simulink model "normal_wave_architecture_constant_passive"  (R2021b)
settings: Solver=ode45  StartTime=0.0  StopTime=20  RelTol=1e-5
values from neighbouring files (symbols this model uses):
  b = 2.1    [normal_wave_architecture_constant_parameters.m]    (also in normal_wave_architecture_constant_parameters.m.m = 8.5; normal_wave_architecture_variable_parameters.m = 1; obs_m.m = block.InputPort(3).Data; obs_s.m = block.InputPort(3).Data)
  Be = 5    [normal_wave_architecture_constant_parameters.m]    (also in normal_wave_architecture_constant_parameters.m.m; normal_wave_architecture_variable_parameters.m)
  beta_m = 2*pi*Fc_vel*Ts    (= 0.0628318530718)    [normal_wave_architecture_constant_parameters.m]    (also in normal_wave_architecture_constant_parameters.m.m; normal_wave_architecture_variable_parameters.m)
  beta_s = 2*pi*Fc_vel*Ts    (= 0.0628318530718)    [normal_wave_architecture_constant_parameters.m]    (also in normal_wave_architecture_constant_parameters.m.m; normal_wave_architecture_variable_parameters.m)
  Bh = 0.02    [normal_wave_architecture_constant_parameters.m]    (also in normal_wave_architecture_constant_parameters.m.m; normal_wave_architecture_variable_parameters.m)
  d_m2s = 1    [normal_wave_architecture_constant_parameters.m]    (also in normal_wave_architecture_constant_parameters.m.m = 10; normal_wave_architecture_variable_parameters.m = 0.001)
  d_s2m = 1    [normal_wave_architecture_constant_parameters.m]    (also in normal_wave_architecture_constant_parameters.m.m = 10; normal_wave_architecture_variable_parameters.m = 0.001)
  delta = 1    [normal_wave_architecture_constant_parameters.m]    (also in normal_wave_architecture_constant_parameters.m.m; normal_wave_architecture_variable_parameters.m)
  eQ_m = 2*pi/4096    (= 0.00153398078789)    [normal_wave_architecture_constant_parameters.m]    (also in normal_wave_architecture_constant_parameters.m.m; normal_wave_architecture_variable_parameters.m)
  eQ_s = 2*pi/4096    (= 0.00153398078789)    [normal_wave_architecture_constant_parameters.m]    (also in normal_wave_architecture_constant_parameters.m.m; normal_wave_architecture_variable_parameters.m)
  Fc_h = 5    [normal_wave_architecture_constant_parameters.m]    (also in normal_wave_architecture_constant_parameters.m.m; normal_wave_architecture_variable_parameters.m)
  Filter = 50    [normal_wave_architecture_constant_parameters.m]    (also in normal_wave_architecture_constant_parameters.m.m = 10; normal_wave_architecture_variable_parameters.m = 1)
  Jh = 0.02    [normal_wave_architecture_constant_parameters.m]    (also in normal_wave_architecture_constant_parameters.m.m; normal_wave_architecture_variable_parameters.m)
  k_m = 19.34    [normal_wave_architecture_constant_parameters.m]    (also in normal_wave_architecture_constant_parameters.m.m; normal_wave_architecture_variable_parameters.m)
  k_s = 19.34    [normal_wave_architecture_constant_parameters.m]    (also in normal_wave_architecture_constant_parameters.m.m; normal_wave_architecture_variable_parameters.m)
  Kc2v_m = 4.5    [normal_wave_architecture_constant_parameters.m]    (also in normal_wave_architecture_constant_parameters.m.m; normal_wave_architecture_variable_parameters.m)
  Kc2v_s = 4.5    [normal_wave_architecture_constant_parameters.m]    (also in normal_wave_architecture_constant_parameters.m.m; normal_wave_architecture_variable_parameters.m)
  Kd_h = 0.5    [normal_wave_architecture_constant_parameters.m]    (also in normal_wave_architecture_constant_parameters.m.m; normal_wave_architecture_variable_parameters.m)
  Kd_m = 0.5    [normal_wave_architecture_constant_parameters.m]    (also in normal_wave_architecture_constant_parameters.m.m; normal_wave_architecture_variable_parameters.m)
  Kd_s = 0.5    [normal_wave_architecture_constant_parameters.m]    (also in normal_wave_architecture_constant_parameters.m.m; normal_wave_architecture_variable_parameters.m)
  Ke = 10    [normal_wave_architecture_constant_parameters.m]    (also in normal_wave_architecture_constant_parameters.m.m; normal_wave_architecture_variable_parameters.m)
  Kp_h = 1.2    [normal_wave_architecture_constant_parameters.m]    (also in normal_wave_architecture_constant_parameters.m.m; normal_wave_architecture_variable_parameters.m)
  Kp_m = 1    [normal_wave_architecture_constant_parameters.m]    (also in normal_wave_architecture_constant_parameters.m.m; normal_wave_architecture_variable_parameters.m)
  Kp_s = 1    [normal_wave_architecture_constant_parameters.m]    (also in normal_wave_architecture_constant_parameters.m.m; normal_wave_architecture_variable_parameters.m)
  Kt2c_m = 1.182    [normal_wave_architecture_constant_parameters.m]    (also in normal_wave_architecture_constant_parameters.m.m; normal_wave_architecture_variable_parameters.m)
  Kt2c_s = 1.182    [normal_wave_architecture_constant_parameters.m]    (also in normal_wave_architecture_constant_parameters.m.m; normal_wave_architecture_variable_parameters.m)
  lArm_m = 0.1    [normal_wave_architecture_constant_parameters.m]    (also in normal_wave_architecture_constant_parameters.m.m; normal_wave_architecture_variable_parameters.m)
  lArm_s = 0.1    [normal_wave_architecture_constant_parameters.m]    (also in normal_wave_architecture_constant_parameters.m.m; normal_wave_architecture_variable_parameters.m)
  qe = 0.5    [normal_wave_architecture_constant_parameters.m]    (also in normal_wave_architecture_constant_parameters.m.m; normal_wave_architecture_variable_parameters.m)
  tau_m = 1.217    [normal_wave_architecture_constant_parameters.m]    (also in normal_wave_architecture_constant_parameters.m.m; normal_wave_architecture_variable_parameters.m)
  tau_s = 1.217    [normal_wave_architecture_constant_parameters.m]    (also in normal_wave_architecture_constant_parameters.m.m; normal_wave_architecture_variable_parameters.m)
  Ts = 0.001    [normal_wave_architecture_constant_parameters.m]    (also in normal_wave_architecture_constant_parameters.m.m; normal_wave_architecture_variable_parameters.m; wave_s.m = Is)
libraries: simulink x2
settings Model: DataTypeOverride=Off  Creator=riccardo  LastModifiedBy=luigi
settings DebuggingCC: IgnoredZcDiagnostic=none  SFMachineParentedDataDiag=warning

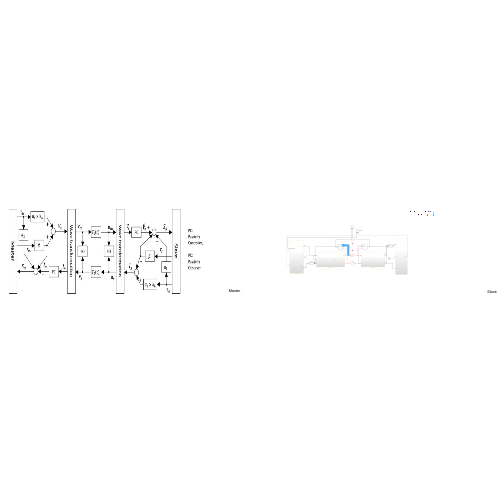
[thumbnail: Simulink's stored preview of the top-level diagram]
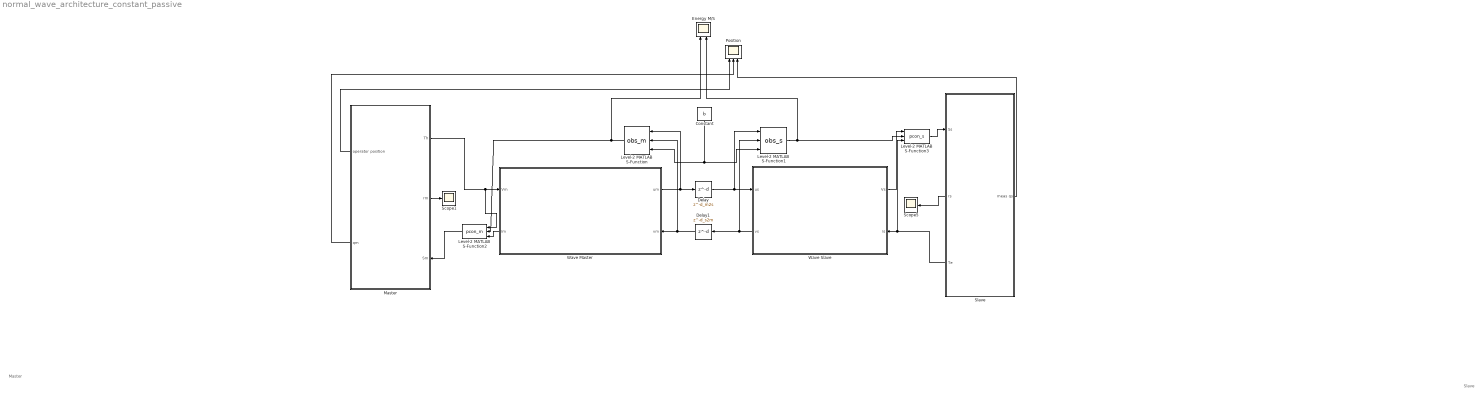
== system normal_wave_architecture_constant_passive ==
  note: Slave
  note: Master
  Constant : Constant  Value=b
  Delay : Delay  DelayLength=d_m2s  SampleTime=Ts
  Delay1 : Delay  DelayLength=d_s2m  SampleTime=Ts
  Energy M/S : Scope  NumInputPorts=2
  Level-2 MATLAB S-Function : M-S-Function  FunctionName=obs_m
  Level-2 MATLAB S-Function1 : M-S-Function  FunctionName=obs_s
  Level-2 MATLAB S-Function2 : M-S-Function  FunctionName=pcon_m
  Level-2 MATLAB S-Function3 : M-S-Function  FunctionName=pcon_s
  Master : Subsystem
      settings: PortSchema="{\"entries\":[{\"content\":{\"sides\":[{\"content\":{\"connectorIds\":[\"Out3\",\"Out4\"]},\"type\":\"ConnectorPlacement.EquallySpacedRectSide\",\"uuid\":\"88a440f3-3c17-4ecd-8a7c-55e312326b6c\"},{\"content\":{\"connectorIds\":[\"Out1\",\"Out2\",\"In1\"],\"side\":\"RIGHT\"},\"type\":\"ConnectorPlacement.EquallySpacedRectSide\",\"uuid\":\"1f119ef7-309b-440c-9250-40a12b2cb029\"},{\"content\":{\"connectorIds\":[],\"side\":\"TOP\"},\"type\":\"ConnectorPlacement.EquallySpacedRectSide\",\"uuid\":\"7be3ae0e-cb45-4f37-96af-a21925a9e765\"}]},\"type\":\"ConnectorPlacement.EquallySpacedConnector\",\"uuid\":\"68cc326c-bdcb-4ff9-98f1-957be474a38c\"}],\"packageUris\":[\"http://schema.mathworks.com/mf0/Connector/R2020b\"],\"version\":\"1.0\"}"
  Position : Scope  NumInputPorts=3
  Scope1 : Scope
  Scope5 : Scope
  Slave : Subsystem
      settings: PortSchema="{\"entries\":[{\"content\":{\"sides\":[{\"content\":{\"connectorIds\":[\"In1\",\"Out2\",\"Out3\"]},\"type\":\"ConnectorPlacement.EquallySpacedRectSide\",\"uuid\":\"d7867d1a-8ca2-46eb-9cc5-3503a790e4da\"},{\"content\":{\"connectorIds\":[\"Out1\"],\"side\":\"RIGHT\"},\"type\":\"ConnectorPlacement.EquallySpacedRectSide\",\"uuid\":\"2f0413cf-eaaa-4002-929a-cebc19c82c9b\"},{\"content\":{\"connectorIds\":[],\"side\":\"TOP\"},\"type\":\"ConnectorPlacement.EquallySpacedRectSide\",\"uuid\":\"f97ed585-16ab-4e7f-97da-40ff87a224f1\"},{\"content\":{\"connectorIds\":[],\"side\":\"BOTTOM\"},\"type\":\"ConnectorPlacement.EquallySpacedRectSide\",\"uuid\":\"e911c9cd-6707-460b-adc0-d2ecc3cf8bb4\"}]},\"type\":\"ConnectorPlacement.EquallySpacedConnector\",\"uuid\":\"a99d57e5-6d89-49cd-b6f9-976c9398d117\"}],\"packageUris\":[\"http://schema.mathworks.com/mf0/Connector/R2020b\"],\"version\":\"1.0\"}"
  Wave Master : Subsystem
      settings: PortSchema="{\"entries\":[{\"content\":{\"sides\":[{\"content\":{\"connectorIds\":[\"In1\",\"Out2\"]},\"type\":\"ConnectorPlacement.EquallySpacedRectSide\",\"uuid\":\"022537ca-6b1a-446a-b70c-5cc8e9763a20\"},{\"content\":{\"connectorIds\":[\"Out1\",\"In2\"],\"side\":\"RIGHT\"},\"type\":\"ConnectorPlacement.EquallySpacedRectSide\",\"uuid\":\"d2fb6654-cfa2-4536-934e-f2f9b55519fe\"},{\"content\":{\"connectorIds\":[],\"side\":\"TOP\"},\"type\":\"ConnectorPlacement.EquallySpacedRectSide\",\"uuid\":\"40d1266d-c1ee-4ea7-83af-e87fd0883292\"}]},\"type\":\"ConnectorPlacement.EquallySpacedConnector\",\"uuid\":\"3d044237-6122-47a2-8c04-12fd83fac9c7\"}],\"packageUris\":[\"http://schema.mathworks.com/mf0/Connector/R2020b\"],\"version\":\"1.0\"}"
  Wave Slave : Subsystem
      settings: PortSchema="{\"entries\":[{\"content\":{\"sides\":[{\"content\":{\"connectorIds\":[\"In1\",\"Out2\"]},\"type\":\"ConnectorPlacement.EquallySpacedRectSide\",\"uuid\":\"022537ca-6b1a-446a-b70c-5cc8e9763a20\"},{\"content\":{\"connectorIds\":[\"Out1\",\"In2\"],\"side\":\"RIGHT\"},\"type\":\"ConnectorPlacement.EquallySpacedRectSide\",\"uuid\":\"d2fb6654-cfa2-4536-934e-f2f9b55519fe\"},{\"content\":{\"connectorIds\":[],\"side\":\"TOP\"},\"type\":\"ConnectorPlacement.EquallySpacedRectSide\",\"uuid\":\"40d1266d-c1ee-4ea7-83af-e87fd0883292\"}]},\"type\":\"ConnectorPlacement.EquallySpacedConnector\",\"uuid\":\"3d044237-6122-47a2-8c04-12fd83fac9c7\"}],\"packageUris\":[\"http://schema.mathworks.com/mf0/Connector/R2020b\"],\"version\":\"1.0\"}"
  wires:
  Slave/1("meas qs ") -> Position/3
  Master/3("operator position ") -> Position/1
  Master/2(rm) -> Scope1/1
  Master/4(qm) -> Position/2
  Slave/2(rs) -> Scope5/1
  Master/1(Th) -> Level-2 MATLAB S-Function2/1, Wave Master/1(Vm)
  Wave Master/1(um) -> Level-2 MATLAB S-Function/1, Delay/1
  Wave Master/2(Im) -> Level-2 MATLAB S-Function2/3
  Delay/1 -> Level-2 MATLAB S-Function1/1, Wave Slave/1(us)
  Slave/3(Te) -> Level-2 MATLAB S-Function3/3, Wave Slave/2(Is)
  Constant/1 -> Level-2 MATLAB S-Function1/3, Level-2 MATLAB S-Function/3
  Delay1/1 -> Level-2 MATLAB S-Function/2, Wave Master/2(vm)
  Level-2 MATLAB S-Function2/1 -> Master/1(Sm)
  Level-2 MATLAB S-Function1/1 -> Energy M/S/2, Level-2 MATLAB S-Function3/2
  Wave Slave/1(Vs) -> Level-2 MATLAB S-Function3/1
  Level-2 MATLAB S-Function3/1 -> Slave/1(Ss)
  Wave Slave/2(vs) -> Level-2 MATLAB S-Function1/2, Delay1/1
  Level-2 MATLAB S-Function/1 -> Level-2 MATLAB S-Function2/2, Energy M/S/1

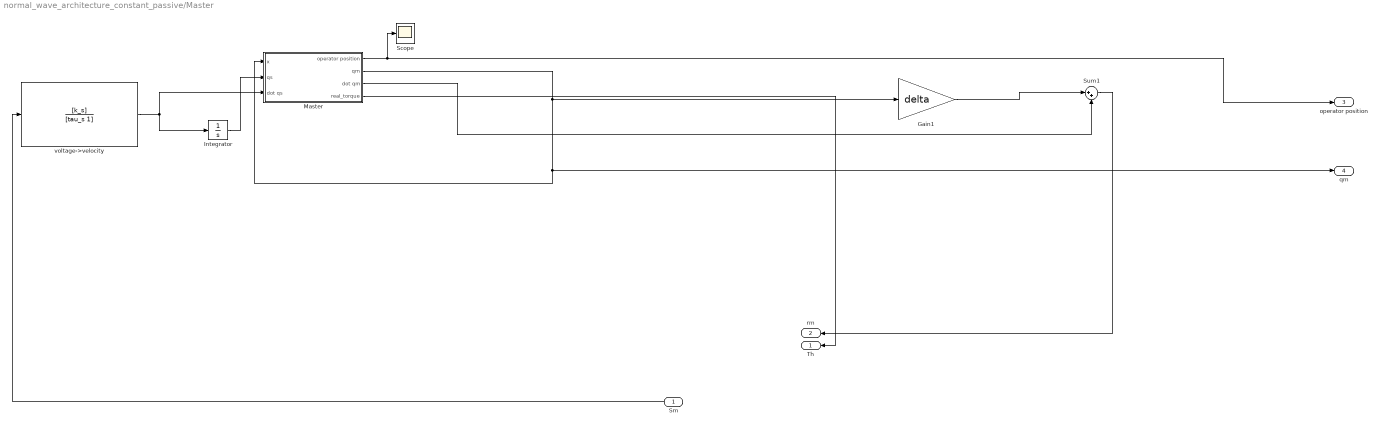
== system normal_wave_architecture_constant_passive/Master ==
  Sm : Inport
  Gain1 : Gain  Gain=delta
  Integrator : Integrator
  Master : Subsystem
  Scope : Scope
  Sum1 : Sum  Inputs=|++
  voltage->velocity : TransferFcn  Numerator=[k_s]  Denominator=[tau_s 1]
  Th : Outport
  rm : Outport  Port=2
  "operator position " : Outport  Port=3
  qm : Outport  Port=4
  wires:
  Master/4(real_torque) -> Th/1
  voltage->velocity/1 -> Master/3(dot qs), Integrator/1
  Gain1/1 -> Sum1/1
  Integrator/1 -> Master/2(qs)
  Master/2(qm) -> Master/1(x), qm/1, Gain1/1
  Master/3(dot qm) -> Sum1/2
  Sm/1 -> voltage->velocity/1
  Master/1("operator position ") -> Scope/1, "operator position "/1
  Sum1/1 -> rm/1

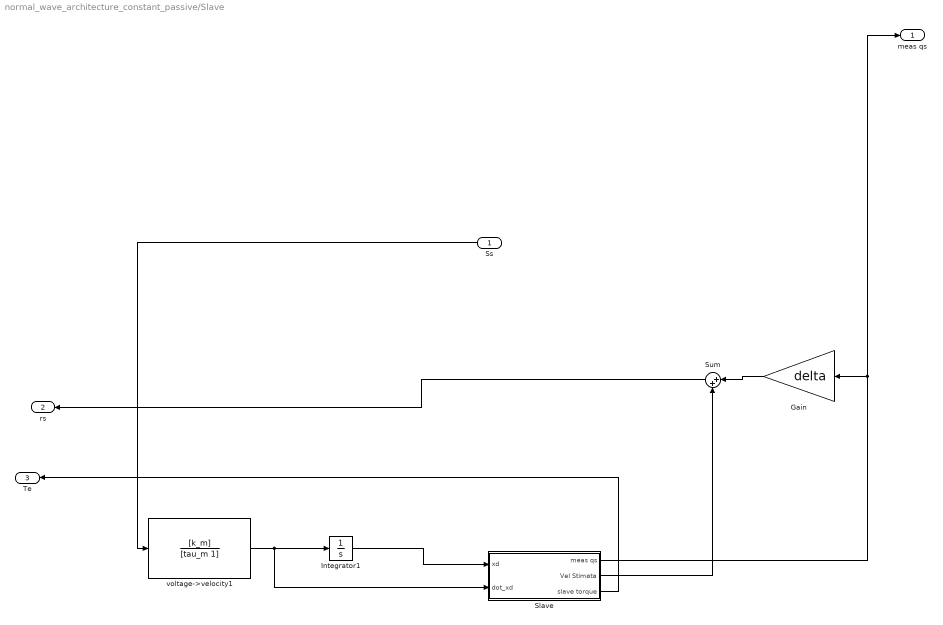
== system normal_wave_architecture_constant_passive/Slave ==
  Ss : Inport
  Gain : Gain  Gain=delta
  Integrator1 : Integrator
  Slave : Subsystem
  Sum : Sum  Inputs=|++
  voltage->velocity1 : TransferFcn  Numerator=[k_m]  Denominator=[tau_m 1]
  "meas qs " : Outport
  rs : Outport  Port=2
  Te : Outport  Port=3
  wires:
  Sum/1 -> rs/1
  Slave/1("meas qs ") -> "meas qs "/1, Gain/1
  Slave/3(slave torque) -> Te/1
  Integrator1/1 -> Slave/1(xd)
  Gain/1 -> Sum/1
  Slave/2("Vel Stimata ") -> Sum/2
  voltage->velocity1/1 -> Integrator1/1, Slave/2(dot_xd)
  Ss/1 -> voltage->velocity1/1

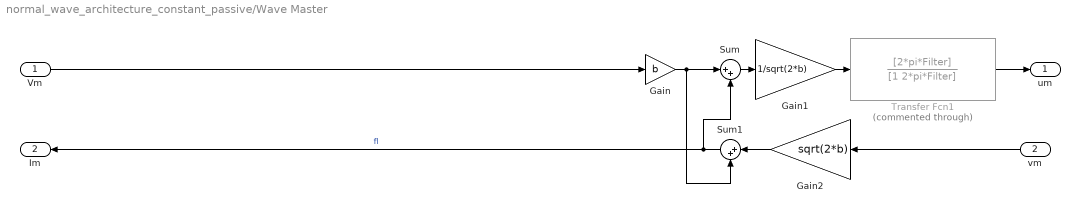
== system normal_wave_architecture_constant_passive/Wave Master ==
  Vm : Inport
  vm : Inport  Port=2
  Gain : Gain  Gain=b
  Gain1 : Gain  Gain=1/sqrt(2*b)
  Gain2 : Gain  Gain=sqrt(2*b)
  Sum : Sum  Inputs=|++
  Sum1 : Sum  Inputs=|++
  Transfer Fcn1 : TransferFcn  Commented=through  Numerator=[2*pi*Filter]  Denominator=[1 2*pi*Filter]
  um : Outport
  Im : Outport  Port=2
  wires:
  Gain/1 -> Sum1/2, Sum/1
  Transfer Fcn1/1 -> um/1
  vm/1 -> Gain2/1
  Gain1/1 -> Transfer Fcn1/1
  Sum/1 -> Gain1/1
  Vm/1 -> Gain/1
  Gain2/1 -> Sum1/1
  Sum1/1 -> Im/1, Sum/2  "fl"

== system normal_wave_architecture_constant_passive/Wave Slave ==
  us : Inport
  Is : Inport  Port=2
  Gain3 : Gain  Gain=sqrt(2*b)
  Gain4 : Gain  Gain=1/b
  Gain5 : Gain  Gain=1/sqrt(2*b)
  Sum2 : Sum  Inputs=|+-
  Sum3 : Sum  Inputs=|+-
  Vs : Outport
  vs : Outport  Port=2
  wires:
  us/1 -> Gain3/1
  Sum2/1 -> Sum3/2, Gain4/1
  Gain3/1 -> Sum2/1
  Is/1 -> Sum2/2, Sum3/1
  Sum3/1 -> Gain5/1
  Gain4/1 -> Vs/1  "dot_xr"
  Gain5/1 -> vs/1

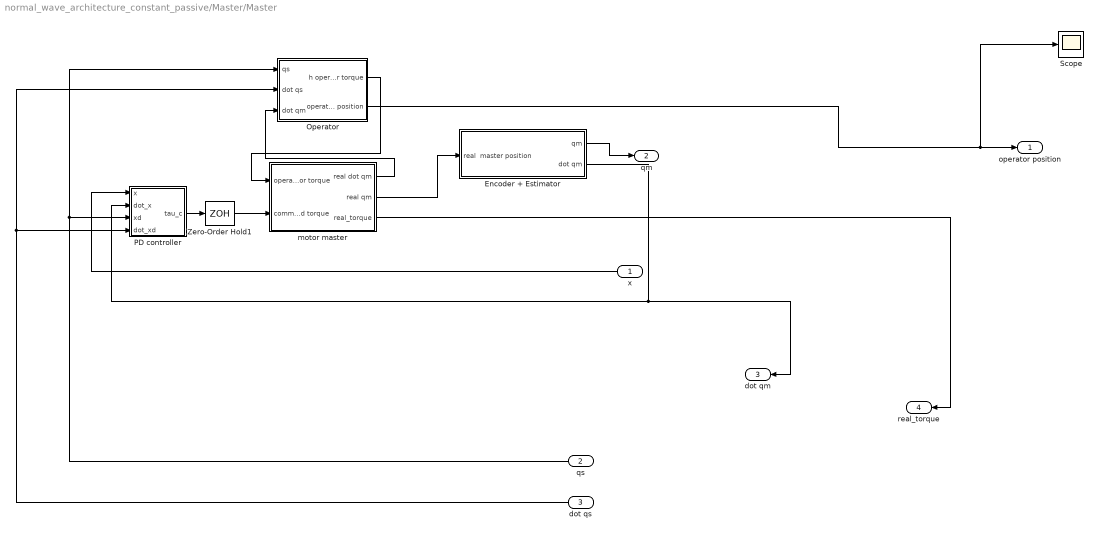
== system normal_wave_architecture_constant_passive/Master/Master ==
  x : Inport
  qs : Inport  Port=2
  dot qs : Inport  Port=3
  Encoder + Estimator : Subsystem
  Operator : Subsystem
  PD controller : Subsystem
  Scope : Scope
  Zero-Order Hold1 : ZeroOrderHold  SampleTime=Ts
  motor master : Subsystem
  "operator position " : Outport
  qm : Outport  Port=2
  dot qm : Outport  Port=3
  real_torque : Outport  Port=4
  wires:
  motor master/1(real dot qm) -> Operator/3(dot qm)
  PD controller/1(tau_c) -> Zero-Order Hold1/1
  qs/1 -> Operator/1(qs), PD controller/3(xd)
  motor master/2(real qm) -> Encoder + Estimator/1(real  master position)
  Operator/1(h operator torque) -> motor master/1(operator torque)
  dot qs/1 -> Operator/2(dot qs), PD controller/4(dot_xd)
  Encoder + Estimator/2(dot qm) -> dot qm/1, PD controller/2(dot_x)
  Encoder + Estimator/1(qm) -> qm/1
  Zero-Order Hold1/1 -> motor master/2(command torque)
  motor master/3(real_torque) -> real_torque/1
  Operator/2("operator position ") -> Scope/1, "operator position "/1
  x/1 -> PD controller/1(x)

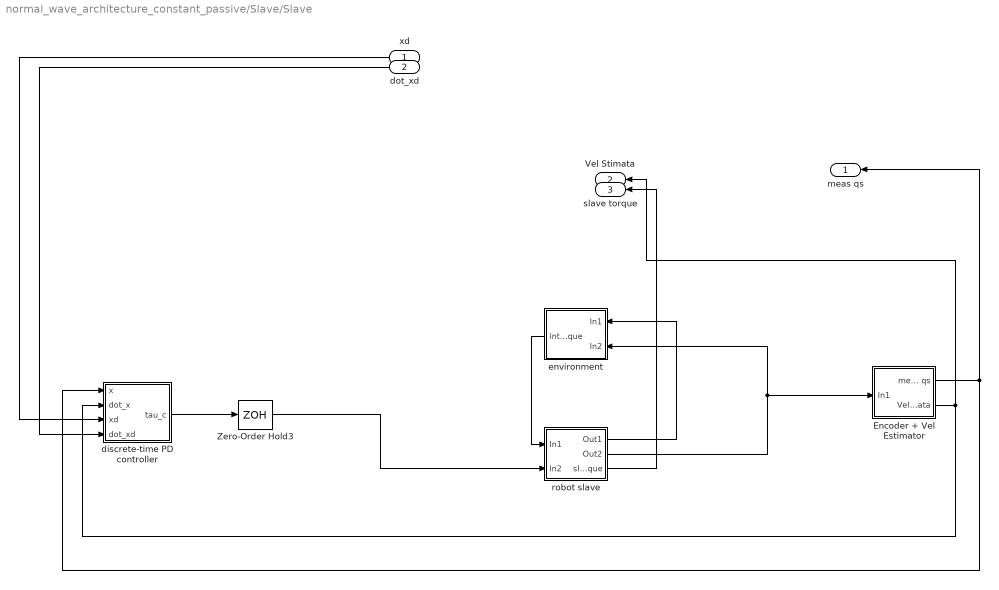
== system normal_wave_architecture_constant_passive/Slave/Slave ==
  xd : Inport
  dot_xd : Inport  Port=2
  "Encoder + Vel Estimator " : Subsystem
  Zero-Order Hold3 : ZeroOrderHold  SampleTime=Ts
  discrete-time PD controller : Subsystem
  "environment " : Subsystem
  "robot slave " : Subsystem
  "meas qs " : Outport
  "Vel Stimata " : Outport  Port=2
  slave torque : Outport  Port=3
  wires:
  "robot slave "/1(Out1) -> "environment "/1(In1)
  "robot slave "/2(Out2) -> "environment "/2(In2), "Encoder + Vel Estimator "/1(In1)
  "Encoder + Vel Estimator "/1("meas qs ") -> "meas qs "/1, discrete-time PD controller/1(x)
  Zero-Order Hold3/1 -> "robot slave "/2(In2)
  "Encoder + Vel Estimator "/2("Vel Stimata ") -> "Vel Stimata "/1, discrete-time PD controller/2(dot_x)
  discrete-time PD controller/1(tau_c) -> Zero-Order Hold3/1
  "environment "/1("interaction torque ") -> "robot slave "/1(In1)
  dot_xd/1 -> discrete-time PD controller/4(dot_xd)
  xd/1 -> discrete-time PD controller/3(xd)
  "robot slave "/3(slave torque) -> slave torque/1

== system normal_wave_architecture_constant_passive/Master/Master/Encoder + Estimator ==
  real  master position : Inport
  Constant : Constant  Value=eQ_m
  Sum : Sum  Inputs=++|
  Velocity estimator : Subsystem
  Zero-Order Hold : ZeroOrderHold  SampleTime=Ts
  noise : MATLAB Function  TreatAsAtomicUnit=on
  qm : Outport
  dot qm : Outport  Port=2
  wires:
  real  master position/1 -> Zero-Order Hold/1
  Zero-Order Hold/1 -> Sum/2
  Sum/1 -> qm/1, Velocity estimator/1(pos misurata)
  Constant/1 -> noise/1(delta_q)
  Velocity estimator/1(Vel stimata) -> dot qm/1
  noise/1(error) -> Sum/1

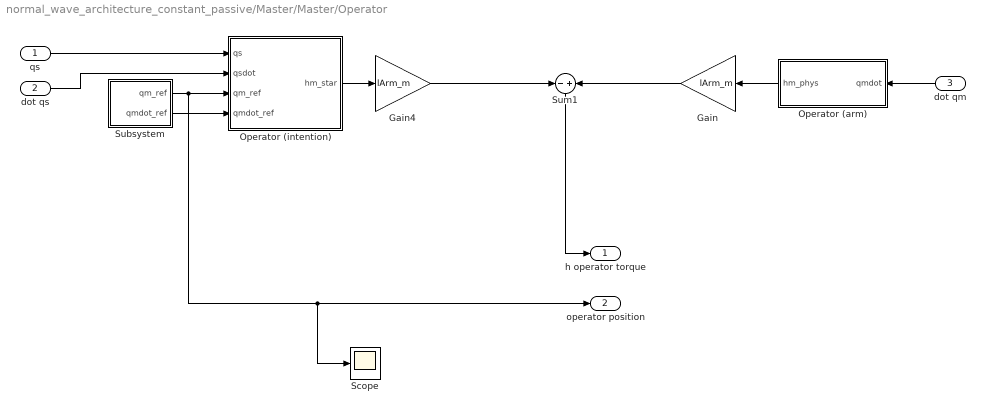
== system normal_wave_architecture_constant_passive/Master/Master/Operator ==
  qs : Inport
  dot qs : Inport  Port=2
  dot qm : Inport  Port=3
  Gain : Gain  Gain=lArm_m
  Gain4 : Gain  Gain=lArm_m
  Operator (arm) : Subsystem
  Operator (intention) : Subsystem
  Scope : Scope
  Subsystem : Subsystem
  Sum1 : Sum  Inputs=-+
  h operator torque : Outport
  "operator position " : Outport  Port=2
  wires:
  Sum1/1 -> h operator torque/1
  Operator (arm)/1(hm_phys) -> Gain/1
  dot qm/1 -> Operator (arm)/1(qmdot)
  Subsystem/2(qmdot_ref) -> Operator (intention)/4(qmdot_ref)
  Operator (intention)/1(hm_star) -> Gain4/1
  dot qs/1 -> Operator (intention)/2(qsdot)
  Gain4/1 -> Sum1/1
  Gain/1 -> Sum1/2
  Subsystem/1(qm_ref) -> Scope/1, "operator position "/1, Operator (intention)/3(qm_ref)
  qs/1 -> Operator (intention)/1(qs)

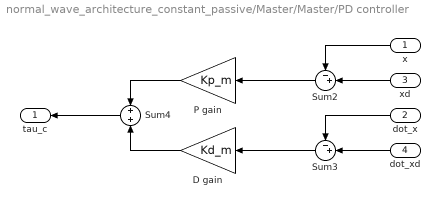
== system normal_wave_architecture_constant_passive/Master/Master/PD controller ==
  x : Inport
  dot_x : Inport  Port=2
  xd : Inport  Port=3
  dot_xd : Inport  Port=4
  D gain : Gain  Gain=Kd_m
  P gain : Gain  Gain=Kp_m
  Sum2 : Sum  Inputs=-+|
  Sum3 : Sum  Inputs=-+|
  Sum4 : Sum
  tau_c : Outport  VectorParamsAs1DForOutWhenUnconnected=off
  wires:
  D gain/1 -> Sum4/2
  dot_x/1 -> Sum3/1
  dot_xd/1 -> Sum3/2
  x/1 -> Sum2/1
  xd/1 -> Sum2/2
  Sum3/1 -> D gain/1
  P gain/1 -> Sum4/1
  Sum4/1 -> tau_c/1
  Sum2/1 -> P gain/1

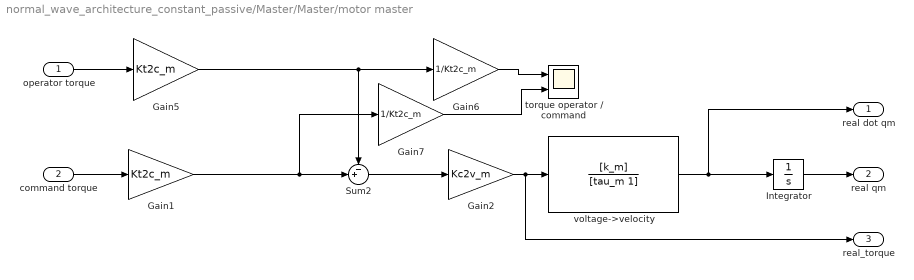
== system normal_wave_architecture_constant_passive/Master/Master/motor master ==
  operator torque : Inport
  command torque : Inport  Port=2
  Gain1 : Gain  Gain=Kt2c_m
  Gain2 : Gain  Gain=Kc2v_m
  Gain5 : Gain  Gain=Kt2c_m
  Gain6 : Gain  Gain=1/Kt2c_m
  Gain7 : Gain  Gain=1/Kt2c_m
  Integrator : Integrator
  Sum2 : Sum  Inputs=-+|
  torque operator / command : Scope  NumInputPorts=2
  voltage->velocity : TransferFcn  Numerator=[k_m]  Denominator=[tau_m 1]
  real dot qm : Outport
  real qm : Outport  Port=2
  real_torque : Outport  Port=3
  wires:
  Gain7/1 -> torque operator / command/2
  operator torque/1 -> Gain5/1
  Gain2/1 -> real_torque/1, voltage->velocity/1
  Gain1/1 -> Gain7/1, Sum2/2
  Integrator/1 -> real qm/1
  command torque/1 -> Gain1/1
  Gain6/1 -> torque operator / command/1
  voltage->velocity/1 -> real dot qm/1, Integrator/1
  Sum2/1 -> Gain2/1
  Gain5/1 -> Sum2/1, Gain6/1

== system normal_wave_architecture_constant_passive/Slave/Slave/Encoder + Vel Estimator  ==
  In1 : Inport
  Constant : Constant  Value=eQ_s
  Subsystem : Subsystem
  Sum : Sum  Inputs=++|
  Zero-Order Hold : ZeroOrderHold  SampleTime=Ts
  noise : MATLAB Function  TreatAsAtomicUnit=on
  "meas qs " : Outport
  "Vel Stimata " : Outport  Port=2
  wires:
  Constant/1 -> noise/1(delta_q)
  In1/1 -> Zero-Order Hold/1
  noise/1(error) -> Sum/1
  Zero-Order Hold/1 -> Sum/2
  Sum/1 -> "meas qs "/1, Subsystem/1(pos misurata)
  Subsystem/1(Vel stimata) -> "Vel Stimata "/1

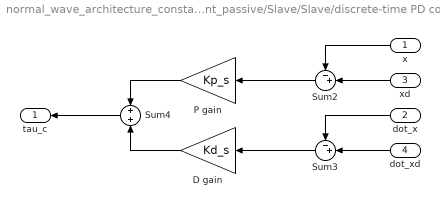
== system normal_wave_architecture_constant_passive/Slave/Slave/discrete-time PD controller ==
  x : Inport
  dot_x : Inport  Port=2
  xd : Inport  Port=3
  dot_xd : Inport  Port=4
  D gain : Gain  Gain=Kd_s
  P gain : Gain  Gain=Kp_s
  Sum2 : Sum  Inputs=-+|
  Sum3 : Sum  Inputs=-+|
  Sum4 : Sum
  tau_c : Outport  VectorParamsAs1DForOutWhenUnconnected=off
  wires:
  D gain/1 -> Sum4/2
  dot_x/1 -> Sum3/1
  dot_xd/1 -> Sum3/2
  x/1 -> Sum2/1
  xd/1 -> Sum2/2
  Sum3/1 -> D gain/1
  P gain/1 -> Sum4/1
  Sum4/1 -> tau_c/1
  Sum2/1 -> P gain/1

== system normal_wave_architecture_constant_passive/Slave/Slave/environment  ==
  note: qs
  note: qdot
  In1 : Inport
  In2 : Inport  Port=2
  Environment : Subsystem
  Gain : Gain  Gain=lArm_s
  "interaction torque " : Outport
  wires:
  In2/1 -> Environment/2(qs)
  Environment/1(fe) -> Gain/1
  In1/1 -> Environment/1(qsdot)
  Gain/1 -> "interaction torque "/1

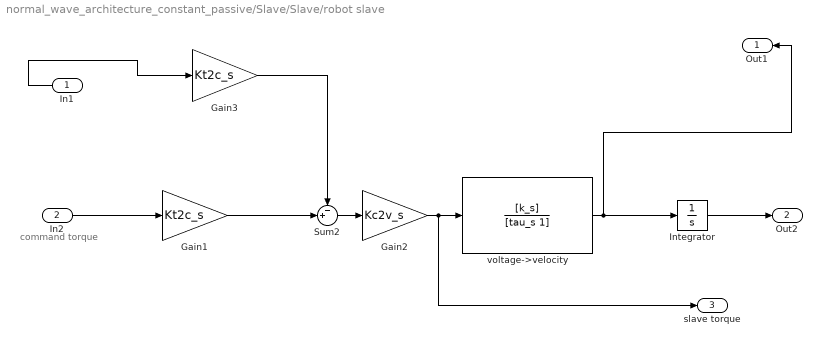
== system normal_wave_architecture_constant_passive/Slave/Slave/robot slave  ==
  note: command torque
  In1 : Inport
  In2 : Inport  Port=2
  Gain1 : Gain  Gain=Kt2c_s
  Gain2 : Gain  Gain=Kc2v_s
  Gain3 : Gain  Gain=Kt2c_s
  Integrator : Integrator
  Sum2 : Sum  Inputs=-+|
  voltage->velocity : TransferFcn  Numerator=[k_s]  Denominator=[tau_s 1]
  Out1 : Outport
  Out2 : Outport  Port=2
  slave torque : Outport  Port=3
  wires:
  Gain2/1 -> slave torque/1, voltage->velocity/1
  Gain3/1 -> Sum2/1
  voltage->velocity/1 -> Out1/1, Integrator/1
  Gain1/1 -> Sum2/2
  Sum2/1 -> Gain2/1
  Integrator/1 -> Out2/1
  In1/1 -> Gain3/1
  In2/1 -> Gain1/1

== system normal_wave_architecture_constant_passive/Master/Master/Encoder + Estimator/Velocity estimator ==
  pos misurata : Inport
  Difference : simulink/Discrete/Difference  ICPrevInput=0.0  OutMin=[]  OutMax=[]  OutDataType=fixdt(1, 16)  OutScaling=2^-10  DoSatur=off
  Filtro passabasso : DiscreteTransferFcn  Numerator=[beta_m 0]  Denominator=[1 -(1-beta_m)]  SampleTime=Ts
  Gain2 : Gain  Gain=1/Ts
  Vel stimata : Outport  VectorParamsAs1DForOutWhenUnconnected=off
  wires:
  Gain2/1 -> Filtro passabasso/1
  pos misurata/1 -> Difference/1
  Difference/1 -> Gain2/1
  Filtro passabasso/1 -> Vel stimata/1  "Velocità  stimata"

== system normal_wave_architecture_constant_passive/Master/Master/Operator/Operator (arm) ==
  note: force
  qmdot : Inport
  Derivative : Derivative  CoefficientInTFapproximation=0.001
  Gain1 : Gain  Gain=Jh
  Gain2 : Gain  Gain=Bh
  Sum : Sum  Inputs=+|+
  hm_phys : Outport  VectorParamsAs1DForOutWhenUnconnected=off
  wires:
  qmdot/1 -> Gain2/1, Derivative/1
  Sum/1 -> hm_phys/1
  Derivative/1 -> Gain1/1
  Gain2/1 -> Sum/1
  Gain1/1 -> Sum/2

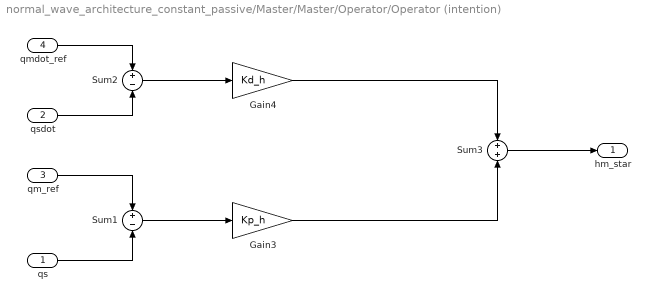
== system normal_wave_architecture_constant_passive/Master/Master/Operator/Operator (intention) ==
  qs : Inport
  qsdot : Inport  Port=2
  qm_ref : Inport  Port=3
  qmdot_ref : Inport  Port=4
  Gain3 : Gain  Gain=Kp_h
  Gain4 : Gain  Gain=Kd_h
  Sum1 : Sum  Inputs=+|-
  Sum2 : Sum  Inputs=+|-
  Sum3 : Sum  Inputs=+|+
  hm_star : Outport  VectorParamsAs1DForOutWhenUnconnected=off
  wires:
  qs/1 -> Sum1/2
  qm_ref/1 -> Sum1/1
  qmdot_ref/1 -> Sum2/1
  Sum1/1 -> Gain3/1
  qsdot/1 -> Sum2/2
  Sum2/1 -> Gain4/1
  Gain4/1 -> Sum3/1
  Gain3/1 -> Sum3/2
  Sum3/1 -> hm_star/1

== system normal_wave_architecture_constant_passive/Master/Master/Operator/Subsystem ==
  Derivative1 : Derivative  CoefficientInTFapproximation=0.001
  Manual Switch : ManualSwitch  CurrentSetting=0
  Sine Wave : Sin  SampleTime=0
  Step : Step  SampleTime=0
  low-pass filter : TransferFcn  Numerator=[2*pi*Fc_h]  Denominator=[1 2*pi*Fc_h]
  qm_ref : Outport
  qmdot_ref : Outport  Port=2
  wires:
  low-pass filter/1 -> Manual Switch/2
  Manual Switch/1 -> qm_ref/1, Derivative1/1
  Derivative1/1 -> qmdot_ref/1  "qmdot_ref"
  Step/1 -> low-pass filter/1
  Sine Wave/1 -> Manual Switch/1

== system normal_wave_architecture_constant_passive/Slave/Slave/Encoder + Vel Estimator /Subsystem ==
  pos misurata : Inport
  Difference : simulink/Discrete/Difference  ICPrevInput=0.0  OutMin=[]  OutMax=[]  OutDataType=fixdt(1, 16)  OutScaling=2^-10  DoSatur=off
  Filtro passabasso : DiscreteTransferFcn  Numerator=[beta_s 0]  Denominator=[1 -(1-beta_s)]  SampleTime=Ts
  Gain2 : Gain  Gain=1/Ts
  Vel stimata : Outport  VectorParamsAs1DForOutWhenUnconnected=off
  wires:
  Gain2/1 -> Filtro passabasso/1
  pos misurata/1 -> Difference/1
  Difference/1 -> Gain2/1
  Filtro passabasso/1 -> Vel stimata/1  "Velocità  stimata"

== system normal_wave_architecture_constant_passive/Slave/Slave/environment /Environment ==
  note: force
  qsdot : Inport
  qs : Inport  Port=2
  Constant : Constant  Value=qe  SampleTime=0
  c1 : Constant  Value=Be  SampleTime=0
  c2 : Constant  Value=Ke  SampleTime=0
  env : MATLAB Function  TreatAsAtomicUnit=on
  fe : Outport  VectorParamsAs1DForOutWhenUnconnected=off
  wires:
  Constant/1 -> env/3(qe)
  c1/1 -> env/2(Be)
  c2/1 -> env/1(Ke)
  qs/1 -> env/4(qs)
  qsdot/1 -> env/5(qsdot)
  env/1(fE) -> fe/1

== matlab function normal_wave_architecture_constant_passive/Slave/Slave/Encoder + Vel Estimator /noise ==
  data: delta_q input; error output
function error = noise_measurement(delta_q)
if randn(1)>0
   error = delta_q;
else
    error = -delta_q;
end

== matlab function normal_wave_architecture_constant_passive/Master/Master/Encoder + Estimator/noise ==
  data: delta_q input; error output
function error = noise_measurement(delta_q)
if randn(1)>0
   error = delta_q;
else
    error = -delta_q;
end

== matlab function normal_wave_architecture_constant_passive/Slave/Slave/environment /Environment/env ==
  data: Ke input; Be input; qe input; qs input; fE output; qsdot input
function fE  = environment(Ke, Be, qe, qs, qsdot)
if qs > qe
   fE = Ke * (qs - qe) + Be * qsdot;
else
   fE = 0;
end
